simulink model "ROTOR"  (R2013a)
settings: Solver=ode45  StartTime=0.0  StopTime=2  RelTol=1e-3
InitFcn:
  | k_d = 1.18e-7
  | B_a = 1.23e-6
  | u_min = 1.25
  | k_t = 3.7e-3
  | k_v = 7.8e-3
  | L_a = 1.9e-3
  | I_G = 1.5e-5
  | R_a = 260e-3
  | m = 0.694
  | l_a = 0.18
  | I_x = 5.87e-3
  | I_y = 5.87e-3
  | I_z = 10.73e-3
libraries: cstblocks x8
settings Model: Creator=root  LastModifiedBy=root

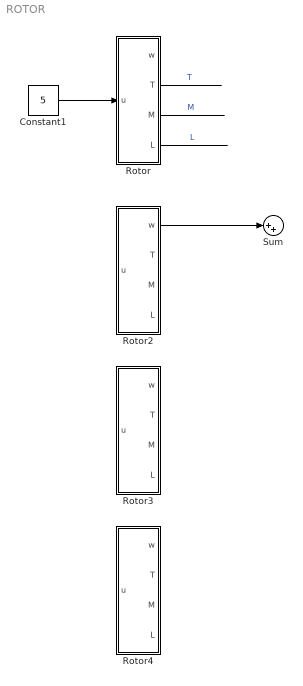
== system ROTOR ==
  Constant1 : Constant  Value=5
  Rotor : Subsystem
  Rotor2 : Subsystem
  Rotor3 : Subsystem
  Rotor4 : Subsystem
  Sum : Sum  Inputs=|++
  wires:
  Constant1/1 -> Rotor/1(u)
  Rotor/2(T) -> ?  "T"
  Rotor/3(M) -> ?  "M"
  Rotor/4(L) -> ?  "L"
  Rotor2/1(w) -> Sum/1

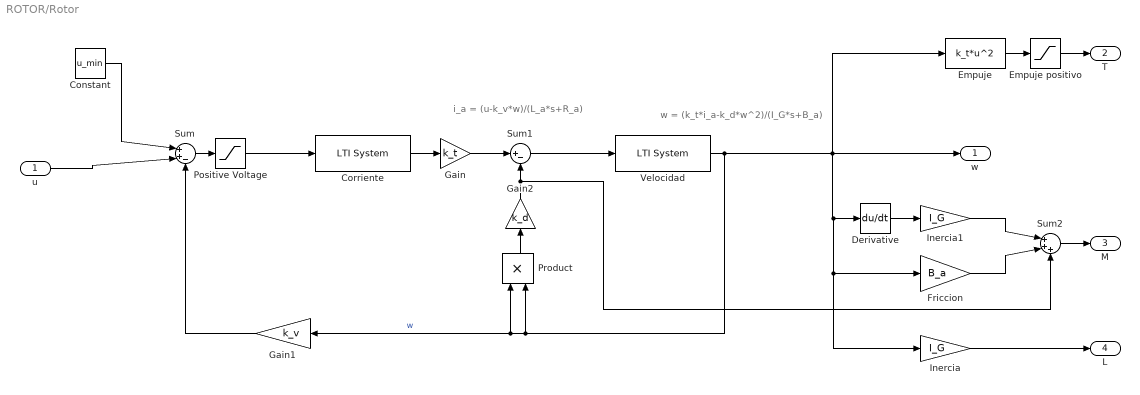
== system ROTOR/Rotor ==
  note: w = (k_t*i_a-k_d*w^2)/(I_G*s+B_a)
  note: i_a = (u-k_v*w)/(L_a*s+R_a)
  u : Inport
  Constant : Constant  Value=u_min
  Corriente : cstblocks/LTI System  sys=tf(1,[L_a R_a])  IC=[]
  Derivative : Derivative
  Empuje : Fcn  Expr=k_t*u^2
  Empuje positivo : Saturate  UpperLimit=inf  LowerLimit=0
  Friccion : Gain  Gain=B_a
  Gain : Gain  Gain=k_t
  Gain1 : Gain  Gain=k_v
  Gain2 : Gain  Gain=k_d
  Inercia : Gain  Gain=I_G
  Inercia1 : Gain  Gain=I_G
  Positive Voltage : Saturate  UpperLimit=30  LowerLimit=0
  Product : Product
  Sum : Sum  Inputs=|++-
  Sum1 : Sum  Inputs=|+-
  Sum2 : Sum  Inputs=|+++
  Velocidad : cstblocks/LTI System  sys=tf(1,[I_G B_a])  IC=[]
  w : Outport
  T : Outport  Port=2
  M : Outport  Port=3
  L : Outport  Port=4
  wires:
  Gain2/1 -> Sum2/3, Sum1/2
  Gain1/1 -> Sum/3
  Velocidad/1 -> Inercia/1, Friccion/1, Derivative/1, Empuje/1, w/1, Product/2, Product/1, Gain1/1  "w"
  u/1 -> Sum/2
  Corriente/1 -> Gain/1
  Sum1/1 -> Velocidad/1
  Product/1 -> Gain2/1
  Sum/1 -> Positive Voltage/1
  Constant/1 -> Sum/1
  Positive Voltage/1 -> Corriente/1
  Gain/1 -> Sum1/1
  Empuje/1 -> Empuje positivo/1
  Empuje positivo/1 -> T/1
  Derivative/1 -> Inercia1/1
  Inercia1/1 -> Sum2/1
  Friccion/1 -> Sum2/2
  Sum2/1 -> M/1
  Inercia/1 -> L/1

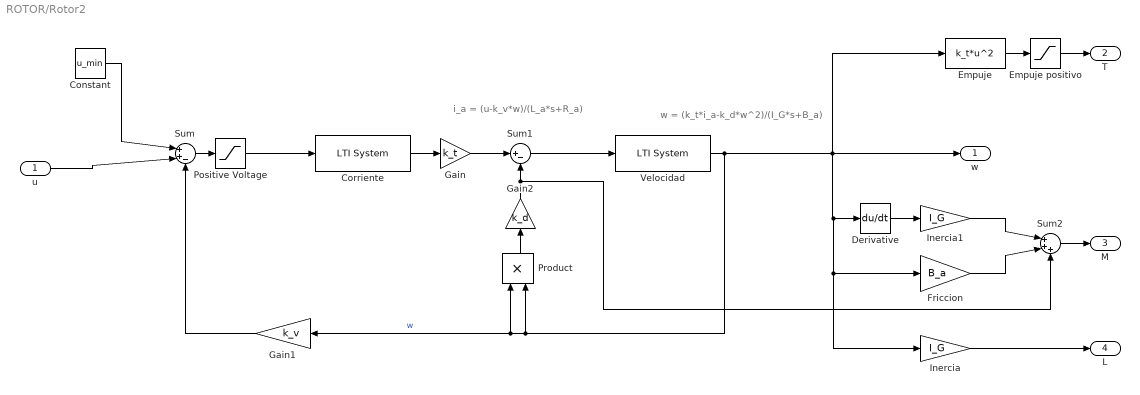
== system ROTOR/Rotor2 ==
  note: i_a = (u-k_v*w)/(L_a*s+R_a)
  note: w = (k_t*i_a-k_d*w^2)/(I_G*s+B_a)
  u : Inport
  Constant : Constant  Value=u_min
  Corriente : cstblocks/LTI System  sys=tf(1,[L_a R_a])  IC=[]
  Derivative : Derivative
  Empuje : Fcn  Expr=k_t*u^2
  Empuje positivo : Saturate  UpperLimit=inf  LowerLimit=0
  Friccion : Gain  Gain=B_a
  Gain : Gain  Gain=k_t
  Gain1 : Gain  Gain=k_v
  Gain2 : Gain  Gain=k_d
  Inercia : Gain  Gain=I_G
  Inercia1 : Gain  Gain=I_G
  Positive Voltage : Saturate  UpperLimit=30  LowerLimit=0
  Product : Product
  Sum : Sum  Inputs=|++-
  Sum1 : Sum  Inputs=|+-
  Sum2 : Sum  Inputs=|+++
  Velocidad : cstblocks/LTI System  sys=tf(1,[I_G B_a])  IC=[]
  w : Outport
  T : Outport  Port=2
  M : Outport  Port=3
  L : Outport  Port=4
  wires:
  Inercia/1 -> L/1
  Sum2/1 -> M/1
  Friccion/1 -> Sum2/2
  Inercia1/1 -> Sum2/1
  Derivative/1 -> Inercia1/1
  Empuje positivo/1 -> T/1
  Empuje/1 -> Empuje positivo/1
  Gain/1 -> Sum1/1
  Positive Voltage/1 -> Corriente/1
  Constant/1 -> Sum/1
  Sum/1 -> Positive Voltage/1
  Product/1 -> Gain2/1
  Sum1/1 -> Velocidad/1
  Corriente/1 -> Gain/1
  u/1 -> Sum/2
  Velocidad/1 -> Gain1/1, Product/1, Product/2, w/1, Empuje/1, Derivative/1, Friccion/1, Inercia/1  "w"
  Gain1/1 -> Sum/3
  Gain2/1 -> Sum1/2, Sum2/3

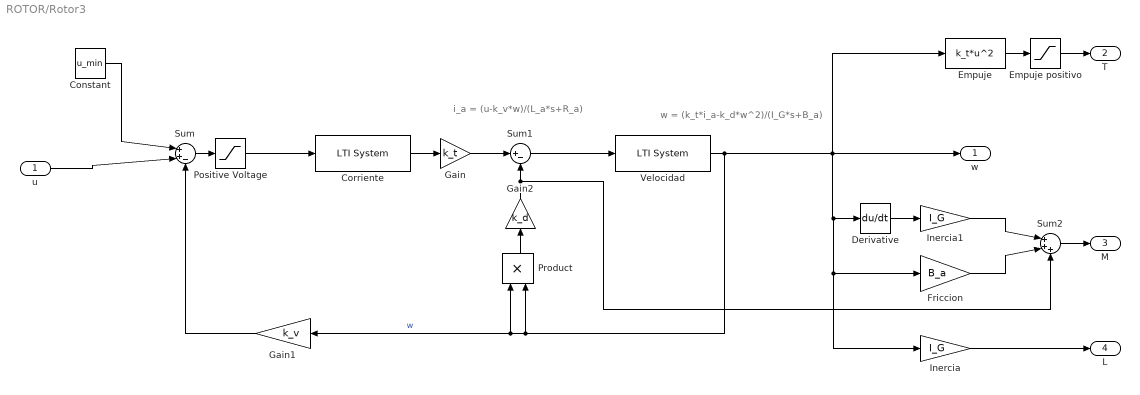
== system ROTOR/Rotor3 ==
  note: w = (k_t*i_a-k_d*w^2)/(I_G*s+B_a)
  note: i_a = (u-k_v*w)/(L_a*s+R_a)
  u : Inport
  Constant : Constant  Value=u_min
  Corriente : cstblocks/LTI System  sys=tf(1,[L_a R_a])  IC=[]
  Derivative : Derivative
  Empuje : Fcn  Expr=k_t*u^2
  Empuje positivo : Saturate  UpperLimit=inf  LowerLimit=0
  Friccion : Gain  Gain=B_a
  Gain : Gain  Gain=k_t
  Gain1 : Gain  Gain=k_v
  Gain2 : Gain  Gain=k_d
  Inercia : Gain  Gain=I_G
  Inercia1 : Gain  Gain=I_G
  Positive Voltage : Saturate  UpperLimit=30  LowerLimit=0
  Product : Product
  Sum : Sum  Inputs=|++-
  Sum1 : Sum  Inputs=|+-
  Sum2 : Sum  Inputs=|+++
  Velocidad : cstblocks/LTI System  sys=tf(1,[I_G B_a])  IC=[]
  w : Outport
  T : Outport  Port=2
  M : Outport  Port=3
  L : Outport  Port=4
  wires:
  Gain2/1 -> Sum2/3, Sum1/2
  Gain1/1 -> Sum/3
  Velocidad/1 -> Inercia/1, Friccion/1, Derivative/1, Empuje/1, w/1, Product/2, Product/1, Gain1/1  "w"
  u/1 -> Sum/2
  Corriente/1 -> Gain/1
  Sum1/1 -> Velocidad/1
  Product/1 -> Gain2/1
  Sum/1 -> Positive Voltage/1
  Constant/1 -> Sum/1
  Positive Voltage/1 -> Corriente/1
  Gain/1 -> Sum1/1
  Empuje/1 -> Empuje positivo/1
  Empuje positivo/1 -> T/1
  Derivative/1 -> Inercia1/1
  Inercia1/1 -> Sum2/1
  Friccion/1 -> Sum2/2
  Sum2/1 -> M/1
  Inercia/1 -> L/1

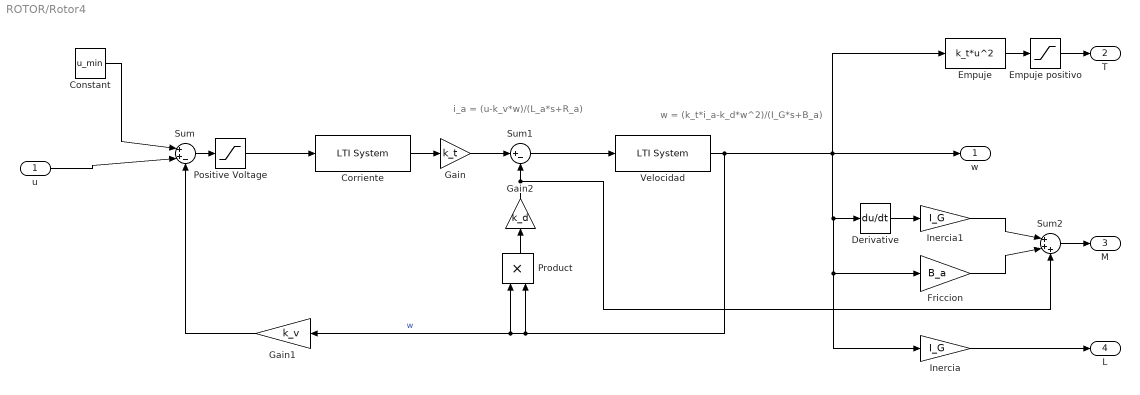
== system ROTOR/Rotor4 ==
  note: i_a = (u-k_v*w)/(L_a*s+R_a)
  note: w = (k_t*i_a-k_d*w^2)/(I_G*s+B_a)
  u : Inport
  Constant : Constant  Value=u_min
  Corriente : cstblocks/LTI System  sys=tf(1,[L_a R_a])  IC=[]
  Derivative : Derivative
  Empuje : Fcn  Expr=k_t*u^2
  Empuje positivo : Saturate  UpperLimit=inf  LowerLimit=0
  Friccion : Gain  Gain=B_a
  Gain : Gain  Gain=k_t
  Gain1 : Gain  Gain=k_v
  Gain2 : Gain  Gain=k_d
  Inercia : Gain  Gain=I_G
  Inercia1 : Gain  Gain=I_G
  Positive Voltage : Saturate  UpperLimit=30  LowerLimit=0
  Product : Product
  Sum : Sum  Inputs=|++-
  Sum1 : Sum  Inputs=|+-
  Sum2 : Sum  Inputs=|+++
  Velocidad : cstblocks/LTI System  sys=tf(1,[I_G B_a])  IC=[]
  w : Outport
  T : Outport  Port=2
  M : Outport  Port=3
  L : Outport  Port=4
  wires:
  Inercia/1 -> L/1
  Sum2/1 -> M/1
  Friccion/1 -> Sum2/2
  Inercia1/1 -> Sum2/1
  Derivative/1 -> Inercia1/1
  Empuje positivo/1 -> T/1
  Empuje/1 -> Empuje positivo/1
  Gain/1 -> Sum1/1
  Positive Voltage/1 -> Corriente/1
  Constant/1 -> Sum/1
  Sum/1 -> Positive Voltage/1
  Product/1 -> Gain2/1
  Sum1/1 -> Velocidad/1
  Corriente/1 -> Gain/1
  u/1 -> Sum/2
  Velocidad/1 -> Gain1/1, Product/1, Product/2, w/1, Empuje/1, Derivative/1, Friccion/1, Inercia/1  "w"
  Gain1/1 -> Sum/3
  Gain2/1 -> Sum1/2, Sum2/3
